simulink model "MODEL_BLOCK"  (R2024b)
settings: Solver=ode45  StartTime=0.0  StopTime=25  FixedStep=0.001  MaxStep=.1  RelTol=1e-3  AbsTol=1e-3
undefined symbols (not defined in the file or in its folder): apf1, apf2, apf4, B1, B2, B3, B4, KI1, KI2, KI4, Kp1, Kp2, Kp3, Kp4, R1, R2, R3, R4, T12, T13, T14, T23, T34, Tg1, Tg2, Tg3, Tg4, Tp1, Tp2, Tp3, Tp4
settings Model: Creator=m2khalaf  LastModifiedBy=amrmo
settings SolverCC: AutoScaleAbsTol=off  AlgebraicLoopSolver=TrustRegion
settings DataIOCC: SaveFormat=Array  SignalLoggingSaveFormat=ModelDataLogs  SaveOutput=off  SaveTime=off  ReturnWorkspaceOutputs=off
settings OptimizationCC: BlockReduction=off  BooleanDataType=off
settings DebuggingCC: SaveWithParameterizedLinksMsg=none  UnderspecifiedInitializationDetection=Classic  MergeDetectMultiDrivingBlocksExec=none  SignalResolutionControl=TryResolveAllWithWarning  MultiTaskDSMMsg=warning  MultiTaskCondExecSysMsg=none  UnconnectedInputMsg=warning  UnconnectedOutputMsg=warning  UnconnectedLineMsg=warning  ArithmeticOperatorsInVariantConditions=warning
settings HardwareCC: TargetUnknown=on
settings ModelReferenceCC: EnableRefExpFcnMdlSchedulingChecks=on  PropagateSignalLabelsOutOfModel=off
settings SFSimCC: SimUseLocalCustomCode=off  CustomCodeUndefinedFunction=UseInterfaceOnly
settings RTWCC: TemplateMakefile=grt_vc.tmf  RTWUseLocalCustomCode=off  GPUComputeCapability=3.5
settings CodeAppCC: StateflowObjectComments=on
settings GRTTargetCC: TargetLangStandard=C89/C90 (ANSI)  CombineOutputUpdateFcns=off  GRTInterface=on

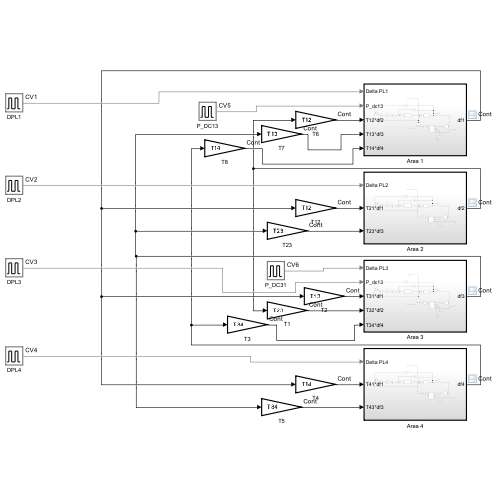
[thumbnail: Simulink's stored preview of the top-level diagram]
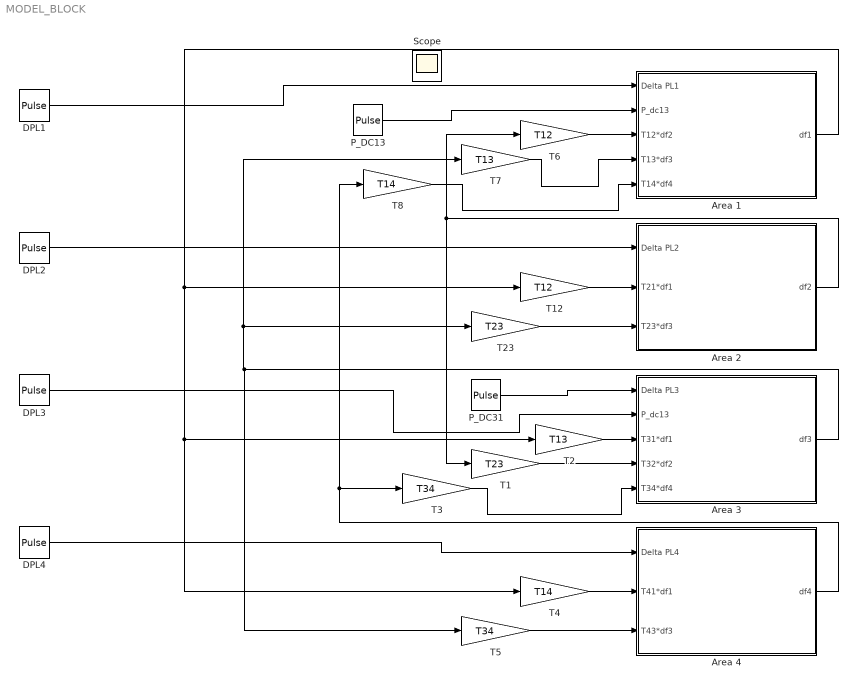
== system MODEL_BLOCK ==
  Area 1 : Subsystem
  Area 2 : Subsystem
  Area 3 : Subsystem
  Area 4 : Subsystem
  DPL1 : DiscretePulseGenerator  PulseType=Time based  Amplitude=0.1  Period=10  PulseWidth=5
  DPL2 : DiscretePulseGenerator  PulseType=Time based  Amplitude=0  Period=10  PulseWidth=5
  DPL3 : DiscretePulseGenerator  PulseType=Time based  Amplitude=0  Period=10  PulseWidth=5
  DPL4 : DiscretePulseGenerator  PulseType=Time based  Amplitude=0  Period=10  PulseWidth=5
  P_DC13 : DiscretePulseGenerator  PulseType=Time based  Amplitude=0  Period=10  PulseWidth=5
  P_DC31 : DiscretePulseGenerator  PulseType=Time based  Amplitude=0  Period=10  PulseWidth=5
  T1 : Gain  Gain=T23  SaturateOnIntegerOverflow=on  OutDataTypeStr=Inherit: Same as input  ParamDataTypeStr=Inherit: Same as input
  T12 : Gain  Gain=T12  SaturateOnIntegerOverflow=on  OutDataTypeStr=Inherit: Same as input  ParamDataTypeStr=Inherit: Same as input
  T2 : Gain  Gain=T13  SaturateOnIntegerOverflow=on  OutDataTypeStr=Inherit: Same as input  ParamDataTypeStr=Inherit: Same as input
  T23 : Gain  Gain=T23  SaturateOnIntegerOverflow=on  OutDataTypeStr=Inherit: Same as input  ParamDataTypeStr=Inherit: Same as input
  T3 : Gain  Gain=T34  SaturateOnIntegerOverflow=on  OutDataTypeStr=Inherit: Same as input  ParamDataTypeStr=Inherit: Same as input
  T4 : Gain  Gain=T14  SaturateOnIntegerOverflow=on  OutDataTypeStr=Inherit: Same as input  ParamDataTypeStr=Inherit: Same as input
  T5 : Gain  Gain=T34  SaturateOnIntegerOverflow=on  OutDataTypeStr=Inherit: Same as input  ParamDataTypeStr=Inherit: Same as input
  T6 : Gain  Gain=T12  SaturateOnIntegerOverflow=on  OutDataTypeStr=Inherit: Same as input  ParamDataTypeStr=Inherit: Same as input
  T7 : Gain  Gain=T13  SaturateOnIntegerOverflow=on  OutDataTypeStr=Inherit: Same as input  ParamDataTypeStr=Inherit: Same as input
  T8 : Gain  Gain=T14  SaturateOnIntegerOverflow=on  OutDataTypeStr=Inherit: Same as input  ParamDataTypeStr=Inherit: Same as input
  Scope : Scope
  wires:
  T12/1 -> Area 2/2(T21*df1)
  T23/1 -> Area 2/3(T23*df3)
  T1/1 -> Area 3/4(T32*df2)
  T2/1 -> Area 3/3(T31*df1)
  T3/1 -> Area 3/5(T34*df4)
  T6/1 -> Area 1/3(T12*df2)
  T7/1 -> Area 1/4(T13*df3)
  T8/1 -> Area 1/5(T14*df4)
  Area 2/1(df2) -> T1/1, T6/1
  Area 3/1(df3) -> T5/1, T23/1, T7/1
  Area 4/1(df4) -> T3/1, T8/1
  Area 1/1(df1) -> T4/1, T2/1, T12/1
  T4/1 -> Area 4/2(T41*df1)
  T5/1 -> Area 4/3(T43*df3)
  P_DC13/1 -> Area 1/2(P_dc13)
  P_DC31/1 -> Area 3/1(Delta PL3)
  DPL1/1 -> Area 1/1(Delta PL1)
  DPL2/1 -> Area 2/1(Delta PL2)
  DPL3/1 -> Area 3/2(P_dc13)
  DPL4/1 -> Area 4/1(Delta PL4)

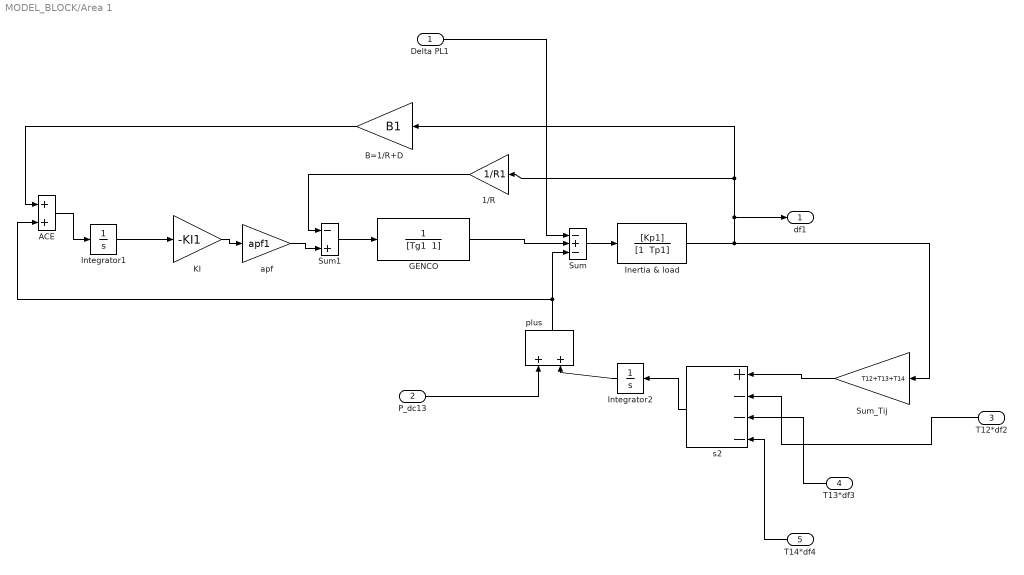
== system MODEL_BLOCK/Area 1 ==
  Delta PL1 : Inport
  P_dc13 : Inport  Port=2
  T12*df2 : Inport  Port=3
  T13*df3 : Inport  Port=4
  T14*df4 : Inport  Port=5
  " GENCO" : TransferFcn  Denominator="[Tg1  1]"  ContinuousStateAttributes='dPm1'
  1/R : Gain  Gain=1/R1  SaturateOnIntegerOverflow=on  OutDataTypeStr=Inherit: Same as input  ParamDataTypeStr=Inherit: Same as input
  ACE : Sum  InputSameDT=on  SaturateOnIntegerOverflow=on  OutDataTypeStr=Inherit: Same as first input
  B=1/R+D : Gain  Gain=B1  SaturateOnIntegerOverflow=on  OutDataTypeStr=Inherit: Same as input  ParamDataTypeStr=Inherit: Same as input
  "Inertia & load " : TransferFcn  Numerator=[Kp1]  Denominator="[1  Tp1]"  ContinuousStateAttributes='df1'
  Integrator1 : Integrator  ContinuousStateAttributes='in1'
  Integrator2 : Integrator  ContinuousStateAttributes='in1'
  KI : Gain  Gain=-KI1  SaturateOnIntegerOverflow=on  OutDataTypeStr=Inherit: Same as input  ParamDataTypeStr=Inherit: Same as input
  Sum : Sum  Inputs=-+-  InputSameDT=on  SaturateOnIntegerOverflow=on  OutDataTypeStr=Inherit: Same as first input
  Sum1 : Sum  Inputs=-+  InputSameDT=on  SaturateOnIntegerOverflow=on  OutDataTypeStr=Inherit: Same as first input
  Sum_Tij : Gain  Gain=T12+T13+T14  SaturateOnIntegerOverflow=on  OutDataTypeStr=Inherit: Same as input  ParamDataTypeStr=Inherit: Same as input
  apf : Gain  Gain=apf1  SaturateOnIntegerOverflow=on  OutDataTypeStr=Inherit: Same as input  ParamDataTypeStr=Inherit: Same as input
  plus : Sum  InputSameDT=on  SaturateOnIntegerOverflow=on  OutDataTypeStr=Inherit: Same as first input
  s2 : Sum  Inputs=+---  InputSameDT=on  SaturateOnIntegerOverflow=on  OutDataTypeStr=Inherit: Same as first input
  df1 : Outport
  wires:
  "Inertia & load "/1 -> B=1/R+D/1, 1/R/1, df1/1, Sum_Tij/1
  B=1/R+D/1 -> ACE/1
  ACE/1 -> Integrator1/1
  1/R/1 -> Sum1/1
  Sum/1 -> "Inertia & load "/1
  " GENCO"/1 -> Sum/2
  Delta PL1/1 -> Sum/1
  Sum1/1 -> " GENCO"/1
  Integrator1/1 -> KI/1
  apf/1 -> Sum1/2
  KI/1 -> apf/1
  plus/1 -> ACE/2, Sum/3
  P_dc13/1 -> plus/1
  Sum_Tij/1 -> s2/1
  s2/1 -> Integrator2/1
  Integrator2/1 -> plus/2
  T12*df2/1 -> s2/2
  T13*df3/1 -> s2/3
  T14*df4/1 -> s2/4

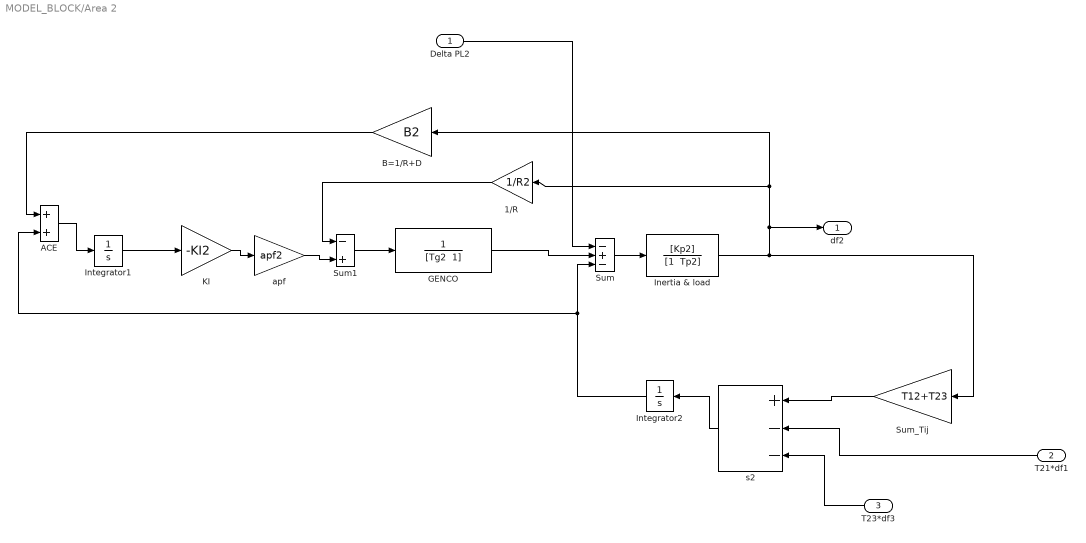
== system MODEL_BLOCK/Area 2 ==
  Delta PL2 : Inport
  T21*df1 : Inport  Port=2
  T23*df3 : Inport  Port=3
  " GENCO" : TransferFcn  Denominator="[Tg2  1]"  ContinuousStateAttributes='dPm2'
  1/R : Gain  Gain=1/R2  SaturateOnIntegerOverflow=on  OutDataTypeStr=Inherit: Same as input  ParamDataTypeStr=Inherit: Same as input
  ACE : Sum  InputSameDT=on  SaturateOnIntegerOverflow=on  OutDataTypeStr=Inherit: Same as first input
  B=1/R+D : Gain  Gain=B2  SaturateOnIntegerOverflow=on  OutDataTypeStr=Inherit: Same as input  ParamDataTypeStr=Inherit: Same as input
  "Inertia & load " : TransferFcn  Numerator=[Kp2]  Denominator="[1  Tp2]"  ContinuousStateAttributes='df2'
  Integrator1 : Integrator  ContinuousStateAttributes='in1'
  Integrator2 : Integrator  ContinuousStateAttributes='in1'
  KI : Gain  Gain=-KI2  SaturateOnIntegerOverflow=on  OutDataTypeStr=Inherit: Same as input  ParamDataTypeStr=Inherit: Same as input
  Sum : Sum  Inputs=-+-  InputSameDT=on  SaturateOnIntegerOverflow=on  OutDataTypeStr=Inherit: Same as first input
  Sum1 : Sum  Inputs=-+  InputSameDT=on  SaturateOnIntegerOverflow=on  OutDataTypeStr=Inherit: Same as first input
  Sum_Tij : Gain  Gain=T12+T23  SaturateOnIntegerOverflow=on  OutDataTypeStr=Inherit: Same as input  ParamDataTypeStr=Inherit: Same as input
  apf : Gain  Gain=apf2  SaturateOnIntegerOverflow=on  OutDataTypeStr=Inherit: Same as input  ParamDataTypeStr=Inherit: Same as input
  s2 : Sum  Inputs=+--  InputSameDT=on  SaturateOnIntegerOverflow=on  OutDataTypeStr=Inherit: Same as first input
  df2 : Outport
  wires:
  "Inertia & load "/1 -> B=1/R+D/1, 1/R/1, df2/1, Sum_Tij/1
  B=1/R+D/1 -> ACE/1
  ACE/1 -> Integrator1/1
  1/R/1 -> Sum1/1
  Sum/1 -> "Inertia & load "/1
  " GENCO"/1 -> Sum/2
  Delta PL2/1 -> Sum/1
  Sum1/1 -> " GENCO"/1
  Integrator1/1 -> KI/1
  apf/1 -> Sum1/2
  KI/1 -> apf/1
  Integrator2/1 -> ACE/2, Sum/3
  Sum_Tij/1 -> s2/1
  s2/1 -> Integrator2/1
  T21*df1/1 -> s2/2
  T23*df3/1 -> s2/3

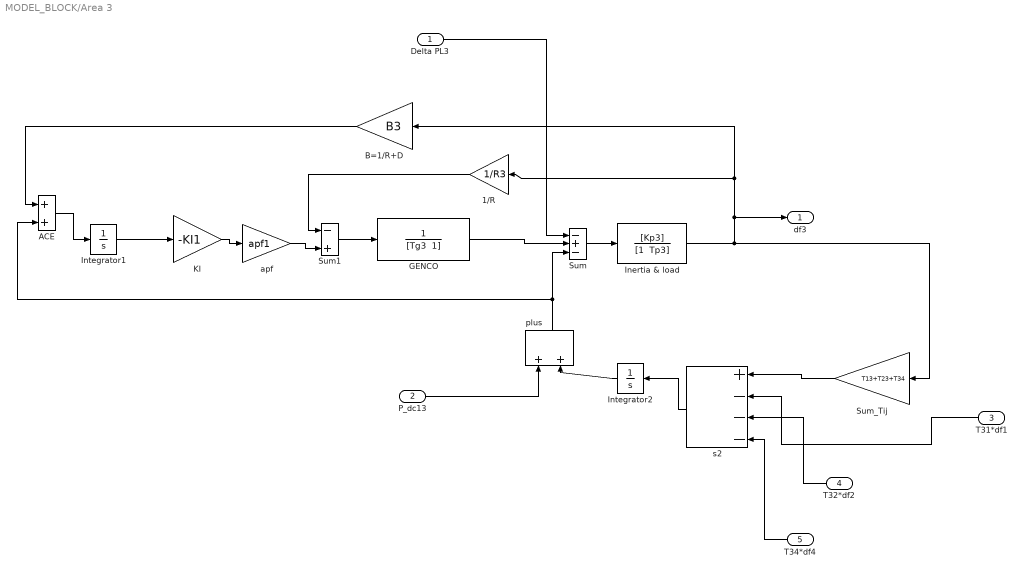
== system MODEL_BLOCK/Area 3 ==
  Delta PL3 : Inport
  P_dc13 : Inport  Port=2
  T31*df1 : Inport  Port=3
  T32*df2 : Inport  Port=4
  T34*df4 : Inport  Port=5
  " GENCO" : TransferFcn  Denominator="[Tg3  1]"  ContinuousStateAttributes='dPm3'
  1/R : Gain  Gain=1/R3  SaturateOnIntegerOverflow=on  OutDataTypeStr=Inherit: Same as input  ParamDataTypeStr=Inherit: Same as input
  ACE : Sum  InputSameDT=on  SaturateOnIntegerOverflow=on  OutDataTypeStr=Inherit: Same as first input
  B=1/R+D : Gain  Gain=B3  SaturateOnIntegerOverflow=on  OutDataTypeStr=Inherit: Same as input  ParamDataTypeStr=Inherit: Same as input
  "Inertia & load " : TransferFcn  Numerator=[Kp3]  Denominator="[1  Tp3]"  ContinuousStateAttributes='df3'
  Integrator1 : Integrator  ContinuousStateAttributes='in1'
  Integrator2 : Integrator  ContinuousStateAttributes='in1'
  KI : Gain  Gain=-KI1  SaturateOnIntegerOverflow=on  OutDataTypeStr=Inherit: Same as input  ParamDataTypeStr=Inherit: Same as input
  Sum : Sum  Inputs=-+-  InputSameDT=on  SaturateOnIntegerOverflow=on  OutDataTypeStr=Inherit: Same as first input
  Sum1 : Sum  Inputs=-+  InputSameDT=on  SaturateOnIntegerOverflow=on  OutDataTypeStr=Inherit: Same as first input
  Sum_Tij : Gain  Gain=T13+T23+T34  SaturateOnIntegerOverflow=on  OutDataTypeStr=Inherit: Same as input  ParamDataTypeStr=Inherit: Same as input
  apf : Gain  Gain=apf1  SaturateOnIntegerOverflow=on  OutDataTypeStr=Inherit: Same as input  ParamDataTypeStr=Inherit: Same as input
  plus : Sum  InputSameDT=on  SaturateOnIntegerOverflow=on  OutDataTypeStr=Inherit: Same as first input
  s2 : Sum  Inputs=+---  InputSameDT=on  SaturateOnIntegerOverflow=on  OutDataTypeStr=Inherit: Same as first input
  df3 : Outport
  wires:
  "Inertia & load "/1 -> B=1/R+D/1, 1/R/1, df3/1, Sum_Tij/1
  B=1/R+D/1 -> ACE/1
  ACE/1 -> Integrator1/1
  1/R/1 -> Sum1/1
  Sum/1 -> "Inertia & load "/1
  " GENCO"/1 -> Sum/2
  Delta PL3/1 -> Sum/1
  Sum1/1 -> " GENCO"/1
  Integrator1/1 -> KI/1
  apf/1 -> Sum1/2
  KI/1 -> apf/1
  plus/1 -> ACE/2, Sum/3
  P_dc13/1 -> plus/1
  Sum_Tij/1 -> s2/1
  s2/1 -> Integrator2/1
  Integrator2/1 -> plus/2
  T31*df1/1 -> s2/2
  T32*df2/1 -> s2/3
  T34*df4/1 -> s2/4

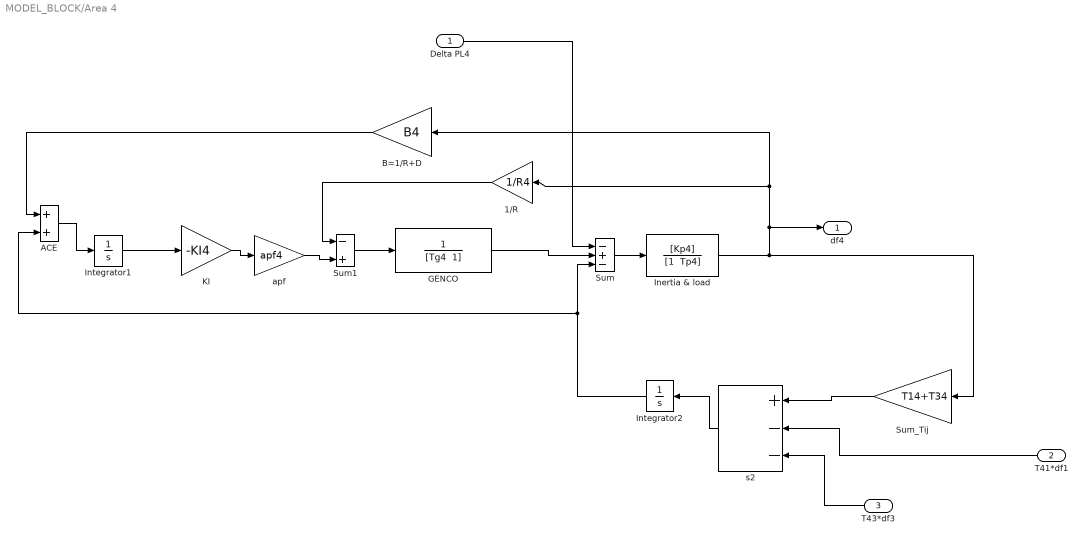
== system MODEL_BLOCK/Area 4 ==
  Delta PL4 : Inport
  T41*df1 : Inport  Port=2
  T43*df3 : Inport  Port=3
  " GENCO" : TransferFcn  Denominator="[Tg4  1]"  ContinuousStateAttributes='dPm4'
  1/R : Gain  Gain=1/R4  SaturateOnIntegerOverflow=on  OutDataTypeStr=Inherit: Same as input  ParamDataTypeStr=Inherit: Same as input
  ACE : Sum  InputSameDT=on  SaturateOnIntegerOverflow=on  OutDataTypeStr=Inherit: Same as first input
  B=1/R+D : Gain  Gain=B4  SaturateOnIntegerOverflow=on  OutDataTypeStr=Inherit: Same as input  ParamDataTypeStr=Inherit: Same as input
  "Inertia & load " : TransferFcn  Numerator=[Kp4]  Denominator="[1  Tp4]"  ContinuousStateAttributes='df4'
  Integrator1 : Integrator  ContinuousStateAttributes='in1'
  Integrator2 : Integrator  ContinuousStateAttributes='in1'
  KI : Gain  Gain=-KI4  SaturateOnIntegerOverflow=on  OutDataTypeStr=Inherit: Same as input  ParamDataTypeStr=Inherit: Same as input
  Sum : Sum  Inputs=-+-  InputSameDT=on  SaturateOnIntegerOverflow=on  OutDataTypeStr=Inherit: Same as first input
  Sum1 : Sum  Inputs=-+  InputSameDT=on  SaturateOnIntegerOverflow=on  OutDataTypeStr=Inherit: Same as first input
  Sum_Tij : Gain  Gain=T14+T34  SaturateOnIntegerOverflow=on  OutDataTypeStr=Inherit: Same as input  ParamDataTypeStr=Inherit: Same as input
  apf : Gain  Gain=apf4  SaturateOnIntegerOverflow=on  OutDataTypeStr=Inherit: Same as input  ParamDataTypeStr=Inherit: Same as input
  s2 : Sum  Inputs=+--  InputSameDT=on  SaturateOnIntegerOverflow=on  OutDataTypeStr=Inherit: Same as first input
  df4 : Outport
  wires:
  "Inertia & load "/1 -> B=1/R+D/1, 1/R/1, df4/1, Sum_Tij/1
  B=1/R+D/1 -> ACE/1
  ACE/1 -> Integrator1/1
  1/R/1 -> Sum1/1
  Sum/1 -> "Inertia & load "/1
  " GENCO"/1 -> Sum/2
  Delta PL4/1 -> Sum/1
  Sum1/1 -> " GENCO"/1
  Integrator1/1 -> KI/1
  apf/1 -> Sum1/2
  KI/1 -> apf/1
  Integrator2/1 -> ACE/2, Sum/3
  Sum_Tij/1 -> s2/1
  s2/1 -> Integrator2/1
  T41*df1/1 -> s2/2
  T43*df3/1 -> s2/3
